simulink model "cable_rob_Magnus"  (R2023b)
settings: Solver=VariableStepAuto  StartTime=0.0  StopTime=T  RelTol=1e-3
InitFcn:
  | run("init_SIM.m")
values from neighbouring files (symbols this model uses):
  R_spool = 0.06    [init_SIM.m]
libraries: slpidlib x4
settings Model: Creator=aamo  LastModifiedBy=magngrot

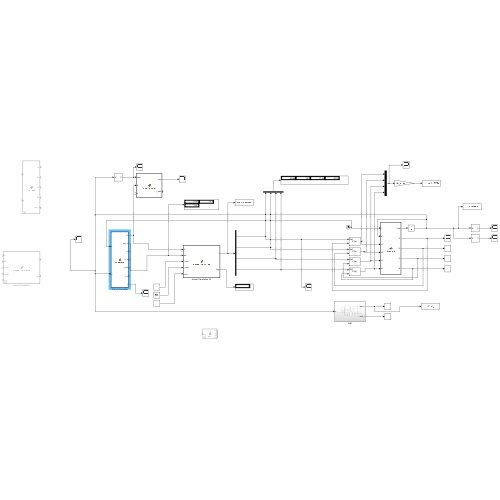
[thumbnail: Simulink's stored preview of the top-level diagram]
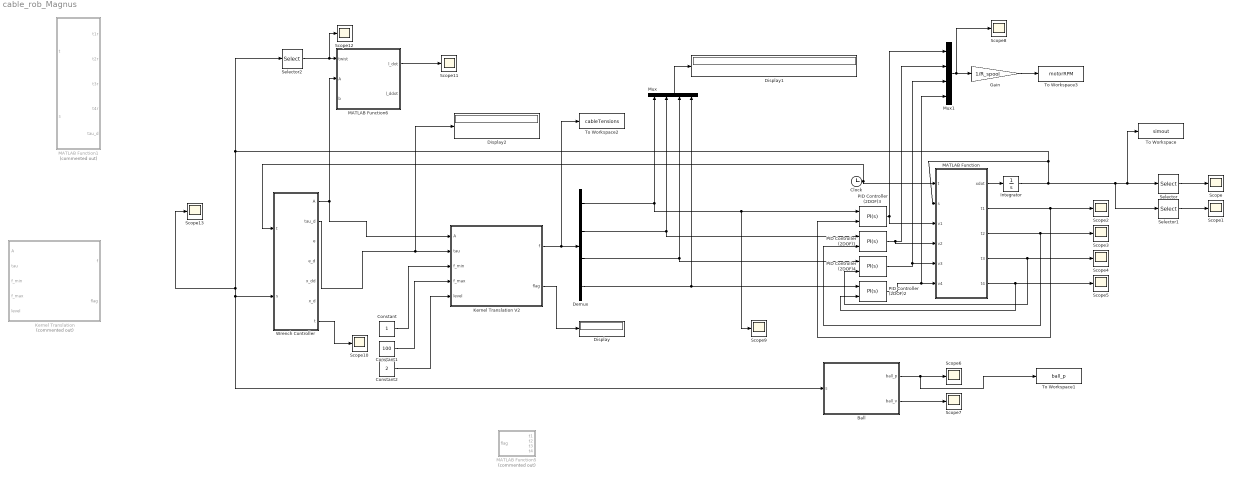
== system cable_rob_Magnus ==
  Ball : Subsystem
  Clock : Clock
  Constant : Constant
  Constant1 : Constant  Value=100
  Constant2 : Constant  Value=2
  Demux : Demux
  Display : Display
  Display1 : Display
  Display2 : Display
  Gain : Gain  Gain=1/R_spool
  Integrator : Integrator  InitialCondition=[0;0;0;0;0;0;1.2039;1.2039;1.2039;1.2039];
  Kernel Translation : MATLAB Function  Commented=on  TreatAsAtomicUnit=on
  Kernel Translation V2 : MATLAB Function  TreatAsAtomicUnit=on
  MATLAB Function : MATLAB Function  TreatAsAtomicUnit=on
  MATLAB Function1 : MATLAB Function  Commented=on  TreatAsAtomicUnit=on
  MATLAB Function5 : MATLAB Function  Commented=on  TreatAsAtomicUnit=on
  MATLAB Function6 : MATLAB Function  TreatAsAtomicUnit=on
  Mux : Mux
  Mux1 : Mux
  PID Controller (2DOF){1..4} (4 alike) : slpidlib/PID Controller (2DOF)  Controller=PI  Form=Parallel  TimeDomain=Continuous-time  UseExternalTs=off  SampleTime=-1  IntegratorMethod=Forward Euler  FilterMethod=Forward Euler  ControllerParametersSource=internal  P=1  I=1  UseKiTs=off  D=1.3  N=100  UseFilter=on  b=1  c=1  TunerSelectOption=Transfer Function Based (PID Tuner App)  InitialConditionSource=internal  InitialConditionForIntegrator=0  InitialConditionForFilter=0  DifferentiatorICPrevScaledInput=0  ExternalReset=none  TrackingMode=off  Kt=1  LimitOutput=off  SatLimitsSource=internal  UpperSaturationLimit=inf  LowerSaturationLimit=-inf  LinearizeAsGain=on  AntiWindupMode=none  Kb=1  LimitIntegrator=off  UpperIntegratorSaturationLimit=inf  LowerIntegratorSaturationLimit=-inf  POutMin=[]  POutMax=[]  IOutMin=[]  IOutMax=[]  DOutMin=[]  DOutMax=[]  NOutMin=[]  NOutMax=[]  bOutMin=[]  bOutMax=[]  cOutMin=[]  cOutMax=[]  SumOutMin=[]  SumOutMax=[]  SaturationOutMin=[]  SaturationOutMax=[]  PParamMin=[]  PParamMax=[]  IParamMin=[]  IParamMax=[]  DParamMin=[]  DParamMax=[]  NParamMin=[]  NParamMax=[]  bParamMin=[]  bParamMax=[]  cParamMin=[]  cParamMax=[]  KbParamMin=[]  KbParamMax=[]  KtParamMin=[]  KtParamMax=[]  KbOutMin=[]  KbOutMax=[]  KtOutMin=[]  KtOutMax=[]  IntegratorOutMin=[]  IntegratorOutMax=[]  FilterOutMin=[]  FilterOutMax=[]  SumI1OutMin=[]  SumI1OutMax=[]  SumI2OutMin=[]  SumI2OutMax=[]  SumI3OutMin=[]  SumI3OutMax=[]  SumI4OutMin=[]  SumI4OutMax=[]  SumDOutMin=[]  SumDOutMax=[]  Sum1OutMin=[]  Sum1OutMax=[]  Sum2OutMin=[]  Sum2OutMax=[]  Sum3OutMin=[]  Sum3OutMax=[]  DifferentiatorOutMin=[]  DifferentiatorOutMax=[]  FilterDiffOutCoefMin=[]  FilterDiffOutCoefMax=[]  ReciprocalOutMin=[]  ReciprocalOutMax=[]  SumDenOutMin=[]  SumDenOutMax=[]  SumNumOutMin=[]  SumNumOutMax=[]  DivideOutMin=[]  DivideOutMax=[]  UdiffTsProdOutMin=[]  UdiffTsProdOutMax=[]  NTsProdOutMin=[]  NTsProdOutMax=[]  UintegralTsProdOutMin=[]  UintegralTsProdOutMax=[]  UngainTsProdOutMin=[]  UngainTsProdOutMax=[]  ClampingZeroOutDataTypeStr=Inherit: Inherit via back propagation  ClampingZeroOutMin=[]  ClampingZeroOutMax=[]  FilterDenConstantOutDataTypeStr=Inherit: Inherit via back propagation  FilterDenConstantOutMin=[]  FilterDenConstantOutMax=[]  PCopyOutDataTypeStr=Inherit: Inherit via back propagation  PCopyOutMin=[]  PCopyOutMax=[]  NCopyOutDataTypeStr=Inherit: Inherit via back propagation  NCopyOutMin=[]  NCopyOutMax=[]  IntegratorContinuousStateAttributes=''  IntegratorStateMustResolveToSignalObject=off  IntegratorRTWStateStorageClass=Auto  FilterContinuousStateAttributes=''  FilterStateMustResolveToSignalObject=off  FilterRTWStateStorageClass=Auto  ParallelPVariant=InternalParameters  IdealPVariant=Disabled  IVariant=InternalParameters  DVariant=Disabled  bVariant=InternalParameters  cVariant=Disabled  IntegratorVariant=Continuous  SatVariant=Disabled  AWVariant=Passthrough  PCopyVariant=Disabled  TRVariant=Disabled  FdbkBlocksVariant=Forward  IdealPFdbkVariant=Disabled  SatFdbkVariant=Disabled  DerivativeFilterVariant=Disabled  NVariant=Disabled  NCopyVariant=Disabled_SignalSpec  FilterICVariant=Disabled  IntegratorICVariant=InternalICs  ExternalResetVariant=Disabled  TRSumVariant=Passthrough  SumFdbkVariant=Disabled  SumVariant=Sum_PI  TsampFilterVariant=InternalTs  TsampNgainVariant=Passthrough  TsampIntegralVariant=Disabled_SignalSpec  ExternalSaturationOutDataTypeStr=Inherit: Same as second input
  Scope{,1..13} (14 alike) : Scope
  Selector : Selector  InputPortWidth=10  IndexOptions=Index vector (dialog)  Indices=[1 2 3]  OutputSizes=1
  Selector1 : Selector  InputPortWidth=10  IndexOptions=Index vector (dialog)  Indices=[7 8 9 10]  OutputSizes=1
  Selector2 : Selector  InputPortWidth=10  IndexOptions=Index vector (dialog)  Indices=[4 5 6]  OutputSizes=1
  To Workspace : ToWorkspace  VariableName=simout  SaveFormat=Timeseries  SampleTime=-1
  To Workspace1 : ToWorkspace  VariableName=ball_p  SaveFormat=Timeseries  SampleTime=-1
  To Workspace2 : ToWorkspace  VariableName=cableTensions  SaveFormat=Timeseries  SampleTime=-1
  To Workspace3 : ToWorkspace  VariableName=motorRPM  SaveFormat=Timeseries  SampleTime=-1
  Wrench Controller : MATLAB Function  TreatAsAtomicUnit=on
  wires:
  MATLAB Function/1(xdot) -> Integrator/1
  Clock/1 -> Wrench Controller/1("t "), MATLAB Function/1(t)
  Integrator/1 -> Selector1/1, To Workspace/1, Selector/1, Wrench Controller/2(s), Ball/1(s), Scope13/1, Selector2/1, MATLAB Function/2(s)
  Selector/1 -> Scope/1
  Selector1/1 -> Scope1/1
  MATLAB Function/2(t1) -> PID Controller (2DOF)3/2, Scope2/1
  PID Controller (2DOF)3/1 -> Mux1/1, MATLAB Function/3(v1)
  Demux/1 -> Scope9/1, PID Controller (2DOF)3/1, Mux/1
  Demux/2 -> PID Controller (2DOF)1/1, Mux/2
  Demux/3 -> PID Controller (2DOF)4/1, Mux/3
  Demux/4 -> PID Controller (2DOF)2/1, Mux/4
  MATLAB Function/3(t2) -> PID Controller (2DOF)1/2, Scope3/1
  MATLAB Function/4(t3) -> PID Controller (2DOF)4/2, Scope4/1
  PID Controller (2DOF)1/1 -> MATLAB Function/4(v2), Mux1/2
  PID Controller (2DOF)4/1 -> Mux1/3, MATLAB Function/5(v3)
  PID Controller (2DOF)2/1 -> Mux1/4, MATLAB Function/6(v4)
  MATLAB Function/5(t4) -> PID Controller (2DOF)2/2, Scope5/1
  Ball/1(ball_p) -> To Workspace1/1, Scope6/1
  Ball/2(ball_v) -> Scope7/1
  Kernel Translation V2/1(f) -> To Workspace2/1, Demux/1
  Kernel Translation V2/2(flag) -> Display/1
  Wrench Controller/2(tau_d) -> Kernel Translation V2/2(tau), Display2/1
  Mux/1 -> Display1/1
  Constant/1 -> Kernel Translation V2/3(f_min)
  Constant1/1 -> Kernel Translation V2/4(f_max)
  Constant2/1 -> Kernel Translation V2/5(level)
  Wrench Controller/1(A) -> Kernel Translation V2/1(A), MATLAB Function6/2(A)
  Mux1/1 -> Scope8/1, Gain/1
  Gain/1 -> To Workspace3/1
  Selector2/1 -> Scope12/1, MATLAB Function6/1(twist)
  MATLAB Function6/1(l_dot) -> Scope11/1
  Wrench Controller/7(t) -> Scope10/1

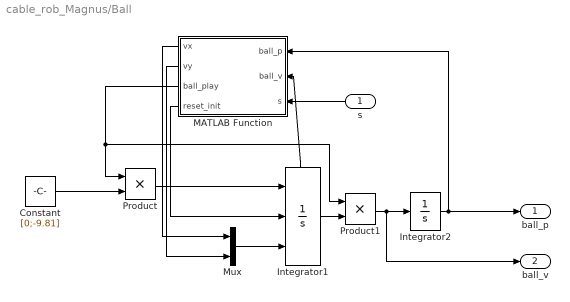
== system cable_rob_Magnus/Ball ==
  s : Inport
  Constant : Constant  Value=[0;-9.81]
  Integrator1 : Integrator  ExternalReset=rising  InitialConditionSource=external  ShowStatePort=on
  Integrator2 : Integrator  InitialCondition=[0;1]
  MATLAB Function : MATLAB Function  TreatAsAtomicUnit=on
  Mux : Mux  Inputs=2
  Product : Product
  Product1 : Product
  ball_p : Outport
  ball_v : Outport  Port=2
  wires:
  Integrator2/1 -> ball_p/1, MATLAB Function/1(ball_p)
  Integrator1/1 -> Product1/2
  Constant/1 -> Product/2
  MATLAB Function/3(ball_play) -> Product/1, Product1/1
  Product/1 -> Integrator1/1
  Integrator1/State -> MATLAB Function/2(ball_v)
  Product1/1 -> ball_v/1, Integrator2/1
  MATLAB Function/4(reset_init) -> Integrator1/2
  s/1 -> MATLAB Function/3(s)
  MATLAB Function/1(vx) -> Mux/1
  MATLAB Function/2(vy) -> Mux/2
  Mux/1 -> Integrator1/3

== matlab function cable_rob_Magnus/MATLAB Function6 ==
  data: twist input; l_dot output; A input; b input; l_ddot output
function [l_dot, l_ddot] = CableDynamics(twist, A, b)
%   xdot:
%      u: matrix of the 4 cable unit vectors
% 

% Velocities and accelerations of the platform
vx = twist(1);
vy = twist(2);
omega = twist(3);    % Angular Velocity
% ax = xdot(4);
% ay = xdot(5);
% alpha = xdot(6);    % Angular Acceleration

% Vector form
v_p = [vx;vy;0];
omega_p = [0;0;omega];
% a_p = [ax;ay;0];
% alpha_p = [0;0;alpha];


% Dynamic Equation by Verhoeven

% % Rate of change of cables
% l_dot = zeros(4,1);
% for i = 1:4
%     b_dot = b_dot_g(v_p, omega_p, psi, b);
%     l_dot(i) = -[u(:,i), 0]'*b_dot;
% end

l_dot = -A*twist;

l_ddot = zeros(4,1);

== matlab function cable_rob_Magnus/Kernel Translation V2 ==
  data: A input; f output; tau input; f_min input; f_max input; level input; flag output
function [f, flag] = KernelTranslation(A,tau,f_min,f_max,level)

[f, flag] = Kernel_translation_ELIAS_V2(A,tau,f_min,f_max,level);

== matlab function cable_rob_Magnus/MATLAB Function1 ==
  settings: updateMethod=DISCRETE
  data: t input; t1r output; s input; t2r output; t3r output; t4r output; tau_d output
function [t1r, t2r, t3r, t4r, tau_d] = controller(t,s)

% Parameters
m = 1;          % Mass of actuator
I = 1;          % Inertia of actuator
length=0.4;     % Horizontal length of actuator
height=0.2;     % Vertical length of actuator
E=100E9;        % Young's modulus of wire
A= 1e-6;        % Cross sectional area of wire

% Anchor points
a1 = [1;1];
a2 = [-1;1];
a3 = [-1;-1];
a4 = [1;-1];

% Position and rotation of actuator
% States
x = s(1); % x-position of actuator
y = s(2); % y-position of actuator
psi = s(3); % rotation of actuator

% Velocities
vx = s(4);
vy = s(5);
vr = s(6);

% Body anchors
b1 = [length/2;height/2];
b2 = [-length/2;height/2];
b3 = [-length/2;-height/2];
b4 = [length/2;-height/2];

% Body anchors in global coordinates
b1g = b_to_g([x;y],psi,b1);
b2g = b_to_g([x;y],psi,b2);
b3g = b_to_g([x;y],psi,b3);
b4g = b_to_g([x;y],psi,b4);

% Length of unstretched cable rolled out.
r1 = s(7);
r2 = s(8);
r3 = s(9);
r4 = s(10);

% Compute tau.
x_d = 0.1*[sin(5*t);
       cos(5*t);
       0];
x_dd = 0.1*[5*cos(5*t);
        -5*sin(5*t);
        0];

% x_d = [0;0;0];
% x_dd = [0;0.2;0];

e = [x;y;psi]-x_d;
e_d = [vx;vy;vr]-x_dd;
D = 10*diag([1,1,1]);
K = 15*diag([5,5,5]);
tau_d = -D*e_d-K*e;

% Compute tenstion setpoints.
%t1r = 20+5*sin(t/4+3);
%t2r = 20+5*sin(t/4+7);
%t3r = 20-5*sin(t/4+2);
%t4r = 20-5*sin(t/4+9);



% Compute force directions
Fd1 = (a1-b1g)/norm(a1-b1g);
Fd2 = (a2-b2g)/norm(a2-b2g);
Fd3 = (a3-b3g)/norm(a3-b3g);
Fd4 = (a4-b4g)/norm(a4-b4g);

% Compute resultant moment
R = [cos(psi), -sin(psi);sin(psi),cos(psi)];
M1 = cross([R*b1;0],[Fd1;0]);
M2 = cross([R*b2;0],[Fd2;0]);
M3 = cross([R*b3;0],[Fd3;0]);
M4 = cross([R*b4;0],[Fd4;0]);


A = [Fd1,Fd2,Fd3,Fd4;
     M1(3), M2(3), M3(3), M4(3)];

tr = pinv(A)*tau_d;

t1r = tr(1);
t2r = tr(2);
t3r = tr(3);
t4r = tr(4);

== matlab function cable_rob_Magnus/MATLAB Function ==
  data: t input; xdot output; s input; t1 output; t2 output; t3 output; t4 output; v1 input; v2 input; v3 input; v4 input
function [xdot,t1,t2,t3,t4] = dynamics(t,s,v1,v2,v3,v4)

% Parameters
m = 1;  % Mass of actuator
I = 1; % Inertia of actuator
length=0.4; % Horizontal length of actuator
height=0.2; % Vertical length of actuator
E=100E9;    % Young's modulus of wire
A= 1e-6;    % Cross sectional area of wire

% Anchor points
a1 = [1;1];
a2 = [-1;1];
a3 = [-1;-1];
a4 = [1;-1];

% Position and rotation of actuator
% States
x = s(1); % x-position of actuator
y = s(2); % y-position of actuator
psi = s(3); % rotation of actuator

% Velocities
vx = s(4);
vy = s(5);
vr = s(6);

% Body anchors
b1 = [length/2;height/2];
b2 = [-length/2;height/2];
b3 = [-length/2;-height/2];
b4 = [length/2;-height/2];

% Body anchors in global coordinates
b1g = b_to_g([x;y],psi,b1);
b2g = b_to_g([x;y],psi,b2);
b3g = b_to_g([x;y],psi,b3);
b4g = b_to_g([x;y],psi,b4);

% Length of unstretched cable rolled out.
r1 = s(7); 
r2 = s(8); 
r3 = s(9); 
r4 = s(10);

% Compute tensions.
t1 = A*E*(norm(b1g-a1) - r1) /r1;
t2 = A*E*(norm(b2g-a2) - r2) /r2;
t3 = A*E*(norm(b3g-a3) - r3) /r3;
t4 = A*E*(norm(b4g-a4) - r4) /r4;

% Compute forces
F1 = t1'*(a1-b1g)/norm(a1-b1g);
F2 = t2'*(a2-b2g)/norm(a2-b2g);
F3 = t3'*(a3-b3g)/norm(a3-b3g);
F4 = t4'*(a4-b4g)/norm(a4-b4g);

% Compute resultant force
F = F1+F2+F3+F4;

% Compute resultant moment
R = [cos(psi), -sin(psi);sin(psi),cos(psi)];
M1 = cross([R*b1;0],[F1;0]);
M2 = cross([R*b2;0],[F2;0]);
M3 = cross([R*b3;0],[F3;0]);
M4 = cross([R*b4;0],[F4;0]);

% Compute resultant moment
M = M1(3)+M2(3)+M3(3)+M4(3);

xdot = [vx;vy;vr;F(1)/m;F(2)/m;M/I;-v1;-v2;-v3;-v4];





% TESTING: direct feedthrough of desired tau.
% xdot = [vx;vy;vr;tau_d(1)/m;tau_d(2)/m;tau_d(3)/I;-v1;-v2;-v3;-v4];

== matlab function cable_rob_Magnus/Ball/MATLAB Function ==
  data: ball_p input; vx output; vy output; ball_play output; ball_v input; reset_init output; s input
function [vx,vy,ball_play,reset_init] = fcn(ball_p,ball_v,s)

length = 0.4;
height = 0.2;

bar_p = s(1:3);
bar_v = s(4:6);

reset_init = 0;

v0 = ball_v;

if ball_p(2)<-1.2 % Ball out of bounds
    v0=[0;0];
    ball_play=0;
    reset_init = 1;
else
    ball_play=1;

    b1 = [length/2;height/2];
    b2 = [-length/2;height/2];

    % Body anchors in global coordinates
    b1g = b_to_g(s(1:2),s(3),b1);
    b2g = b_to_g(s(1:2),s(3),b2);

    if ball_p(2)<=-1
        reset_init=1;
        v0 = diag([1,-0.95])*ball_v; % Just jump off the bottom.
    elseif ball_p(1)>=b2g(1) && ball_p(1)<=b1g(1)  % Ball can potentially cross.
        dy = b1g(2)-b2g(2);
        dx = b1g(1)-b2g(1);
        inc = dy/dx;
        if ball_p(2)<=b2g(2)+inc*(ball_p(1)-b2g(1))
            reset_init=1;
            e_p = (b1g-b2g)/norm(b1g-b2g); % Paralell with bar.
            e_n = [-e_p(2);e_p(1)];        % Normal to bar.
            vip = ball_v'*e_p * e_p;
            vin = ball_v'*e_n * e_n;
            v0 = vip-vin;
        end
    end
end

vx = v0(1);
vy = v0(2);

== matlab function cable_rob_Magnus/Wrench Controller ==
  settings: updateMethod=DISCRETE
  data: A output; t input; s input; tau_d output; e output; e_d output; x_dd output; x_d output; t output
function [A,tau_d, e, e_d, x_dd, x_d, t] = controller(t,s)

% Parameters
m = 0.1;                % Mass of actuator
I = 1;                  % Inertia of actuator
length=0.4;             % Horizontal length of actuator
height=0.2;             % Vertical length of actuator
E=100E9;                % Young's modulus of wire
A_cross= 1e-6;          % Cross sectional area of wire

% Anchor points
a1 = [1;1];
a2 = [-1;1];
a3 = [-1;-1];
a4 = [1;-1];

% Position and rotation of actuator
% States
x = s(1); % x-position of actuator
y = s(2); % y-position of actuator
psi = s(3); % rotation of actuator

% Velocities
vx = s(4);
vy = s(5);
vr = s(6);

% Body anchors
b1 = [length/2;height/2];
b2 = [-length/2;height/2];
b3 = [-length/2;-height/2];
b4 = [length/2;-height/2];

% Body anchors in global coordinates
b1g = b_to_g([x;y],psi,b1);
b2g = b_to_g([x;y],psi,b2);
b3g = b_to_g([x;y],psi,b3);
b4g = b_to_g([x;y],psi,b4);

% Length of unstretched cable rolled out.
r1 = s(7);
r2 = s(8);
r3 = s(9);
r4 = s(10);

% Compute tau.
x_d = 0.5*[sin(5*t);
       cos(5*t);
       0];
x_dd = 0.1*[5*cos(5*t);
        -5*sin(5*t);
        0];

% x_d = [0;0;0];
% x_dd = [0;0.2;0];

e = [x;y;psi]-x_d;
e_d = [vx;vy;vr]-x_dd;

% D = 10*diag([1,1,1]);
% K = 15*diag([5,5,5]);
D = 2*diag([1,1,1]);
K = 6*diag([5,5,5]);
 % tau_d = -D*e_d-K*e;
tau_d = D*e_d+K*e;

% Compute tenstion setpoints.
%t1r = 20+5*sin(t/4+3);
%t2r = 20+5*sin(t/4+7);
%t3r = 20-5*sin(t/4+2);
%t4r = 20-5*sin(t/4+9);



% Compute force directions
Fd1 = (a1-b1g)/norm(a1-b1g);
Fd2 = (a2-b2g)/norm(a2-b2g);
Fd3 = (a3-b3g)/norm(a3-b3g);
Fd4 = (a4-b4g)/norm(a4-b4g);

% Compute resultant moment
R = [cos(psi), -sin(psi);sin(psi),cos(psi)];
M1 = cross([R*b1;0],[Fd1;0]);
M2 = cross([R*b2;0],[Fd2;0]);
M3 = cross([R*b3;0],[Fd3;0]);
M4 = cross([R*b4;0],[Fd4;0]);


A_t = [Fd1,Fd2,Fd3,Fd4;
     M1(3), M2(3), M3(3), M4(3)];

tr = pinv(A_t)*tau_d;

t1r = tr(1);
t2r = tr(2);
t3r = tr(3);
t4r = tr(4);

A = A_t';

== matlab function cable_rob_Magnus/Kernel Translation ==
  data: A input; f output; tau input; f_min input; f_max input; level input; flag output
function [f, flag] = KernelTranslation(A,tau,f_min,f_max,level)

[f, flag] = Kernel_translation_Elias(A,tau,f_min,f_max,level);

== matlab function cable_rob_Magnus/MATLAB Function5 ==
  data: flag input; t1 output; t2 output; t3 output; t4 output
function [t1,t2,t3,t4] = fcn(flag)

y = u;
